simulink model "Waveformmodel"  (R2021a)
settings: Solver=FixedStepAuto  StartTime=0.0  StopTime=1  FixedStep=0.001  RelTol=1e-3
values from neighbouring files (symbols this model uses):
  Clamp1Amp = x(2)    [Opti_Clamp1.m]    (also in Opti_Clamp1_exp.m; Opti_Clamp2.m = 0; Opti_Clamp2_exp.m = 0; Opti_ClampsSine.m = 0)
  Clamp1Width = x(1)    [Opti_Clamp1.m]    (also in Opti_Clamp1_exp.m; Opti_ClampsSine.m = 0.001; Opti_Shears.m = 0.001; Opti_fit_exp.m = 0.001)
  Clamp2Amp = 0    [Opti_Clamp1.m]    (also in Opti_Clamp1_exp.m; Opti_ClampsSine.m; Opti_ClampsSine_exp.m; Opti_Shears.m)
  Clamp2Width = 0.001    [Opti_Clamp1.m]    (also in Opti_Clamp1_exp.m; Opti_ClampsSine_exp.m; Opti_Shears_exp.m; Opti_fit_exp.m)
  ClampsSineAmp = 0    [Opti_Clamp1.m]    (also in Opti_Clamp1_exp.m; Opti_Clamp2.m; Opti_Clamp2_exp.m; Opti_Shears.m)
  ClampsSineWidth = 0.001    [Opti_Clamp1.m]    (also in Opti_Clamp1_exp.m; Opti_Clamp2.m; Opti_Clamp2_exp.m; Opti_Shears.m)
  pAmpGain = 1./[25, 25, 7.5, 7.5]    [Main.m]    (also in Opti_Clamp1.m; Opti_Clamp1_exp.m; Opti_clamp05pi.m; Opti_fit_exp.m)
  pClampAmpl = (pClampMax - pClampMin) / 2    (= 45)    [Main.m]    (also in Opti_Clamp1.m; Opti_Clamp1_exp.m; Opti_clamp05pi.m; Opti_fit_exp.m)
  pClampOffs = (pClampMax + pClampMin) / 2    (= 15)    [Main.m]    (also in Opti_Clamp.m = (pClampMax + pClampMin) / 2; Opti_Clamp1.m; Opti_Clamp1_exp.m; Opti_Clamp2.m = (pClampMax + pClampMin) / 2)
  pClampSatMax = 60    [Main.m]    (also in Opti_Clamp.m; Opti_Clamp1.m; Opti_Clamp1_exp.m; Opti_Clamp2.m)
  pClampSatMin = -30    [Main.m]    (also in Opti_Clamp1.m; Opti_Clamp1_exp.m; Opti_clamp05pi.m; Opti_fit_exp.m)
  pShearAmpl = (pShearMax - pShearMin) / 2    (= 150)    [Main.m]    (also in Opti_Clamp1.m; Opti_Clamp1_exp.m; Opti_clamp05pi.m; Opti_fit_exp.m)
  pShearOffs = (pShearMax + pShearMin) / 2    (= 0)    [Main.m]    (also in Opti_Clamp.m = (pShearMax + pShearMin) / 2; Opti_Clamp1.m; Opti_Clamp1_exp.m; Opti_Clamp2.m = (pShearMax + pShearMin) / 2)
  pShearSatMax = 250    [Main.m]    (also in Opti_Clamp.m; Opti_Clamp1.m; Opti_Clamp1_exp.m; Opti_Clamp2.m)
  pShearSatMin = -250    [Main.m]    (also in Opti_Clamp1.m; Opti_Clamp1_exp.m; Opti_clamp05pi.m; Opti_fit_exp.m)
  ShearAmp = 0    [Opti_Clamp1.m]    (also in Opti_Clamp1_exp.m; Opti_Clamp2.m; Opti_Clamp2_exp.m; Opti_ClampsSine.m)
  ShearWidth = 0.001    [Opti_Clamp1.m]    (also in Opti_Clamp1_exp.m; Opti_Clamp2.m; Opti_Clamp2_exp.m; Opti_ClampsSine.m)
libraries: simulink x2
settings Model: Creator=20191779  LastModifiedBy=20191779

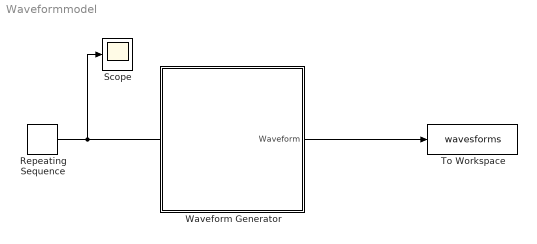
== system Waveformmodel ==
  Repeating Sequence : simulink/Sources/Repeating Sequence  rep_seq_t=[0 1 2]  rep_seq_y=[0 5 0]*5e-6
  Scope : Scope
  To Workspace : ToWorkspace  VariableName=wavesforms  SampleTime=-1
  Waveform Generator : Subsystem
  wires:
  Repeating Sequence/1 -> Scope/1
  Waveform Generator/1(Waveform) -> To Workspace/1

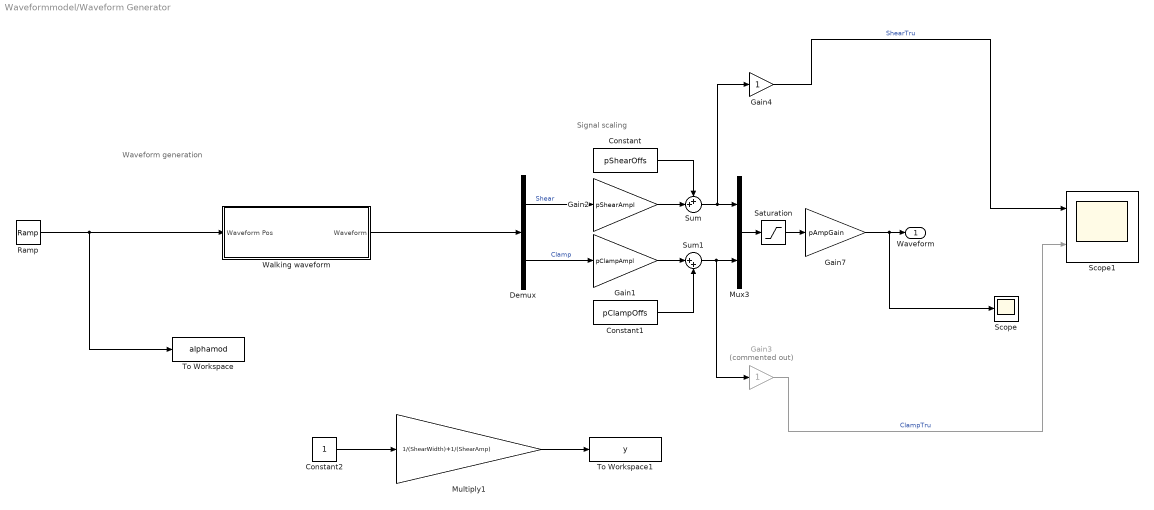
== system Waveformmodel/Waveform Generator ==
  note: Waveform generation
  note: Signal scaling
  Constant : Constant  Value=pShearOffs
  Constant1 : Constant  Value=pClampOffs
  Constant2 : Constant
  Demux : Demux  Outputs=2
  Gain1 : Gain  Gain=pClampAmpl
  Gain2 : Gain  Gain=pShearAmpl
  Gain3 : Gain  Commented=on
  Gain4 : Gain
  Gain7 : Gain  Gain=pAmpGain
  Multiply1 : Gain  Gain=1/(ShearWidth)+1/(ShearAmp)
  Mux3 : Mux  Inputs=2
  Ramp : simulink/Sources/Ramp  slope=2*pi  start=0  InitialOutput=0
  Saturation : Saturate  UpperLimit=[pShearSatMax pShearSatMax pClampSatMax pClampSatMax]  LowerLimit=[pShearSatMin pShearSatMin pClampSatMin pClampSatMin]
  Scope : Scope
  Scope1 : Scope  NumInputPorts=2
  Sum : Sum  Inputs=++|
  Sum1 : Sum  Inputs=|++
  To Workspace : ToWorkspace  VariableName=alphamod  SampleTime=-1
  To Workspace1 : ToWorkspace  VariableName=y  SampleTime=-1
  Walking waveform : Subsystem  TreatAsAtomicUnit=on
  Waveform : Outport  VectorParamsAs1DForOutWhenUnconnected=off
  wires:
  Gain2/1 -> Sum/2
  Constant/1 -> Sum/1
  Gain1/1 -> Sum1/1
  Constant1/1 -> Sum1/2
  Demux/1 -> Gain2/1  "Shear"
  Demux/2 -> Gain1/1  "Clamp"
  Gain3/1 -> Scope1/2  "ClampTru"
  Gain4/1 -> Scope1/1  "ShearTru"
  Walking waveform/1(Waveform) -> Demux/1
  Mux3/1 -> Saturation/1
  Gain7/1 -> Scope/1, Waveform/1
  Sum/1 -> Gain4/1, Mux3/1
  Sum1/1 -> Gain3/1, Mux3/2
  Saturation/1 -> Gain7/1
  Ramp/1 -> To Workspace/1, Walking waveform/1(Waveform Pos)
  Constant2/1 -> Multiply1/1
  Multiply1/1 -> To Workspace1/1

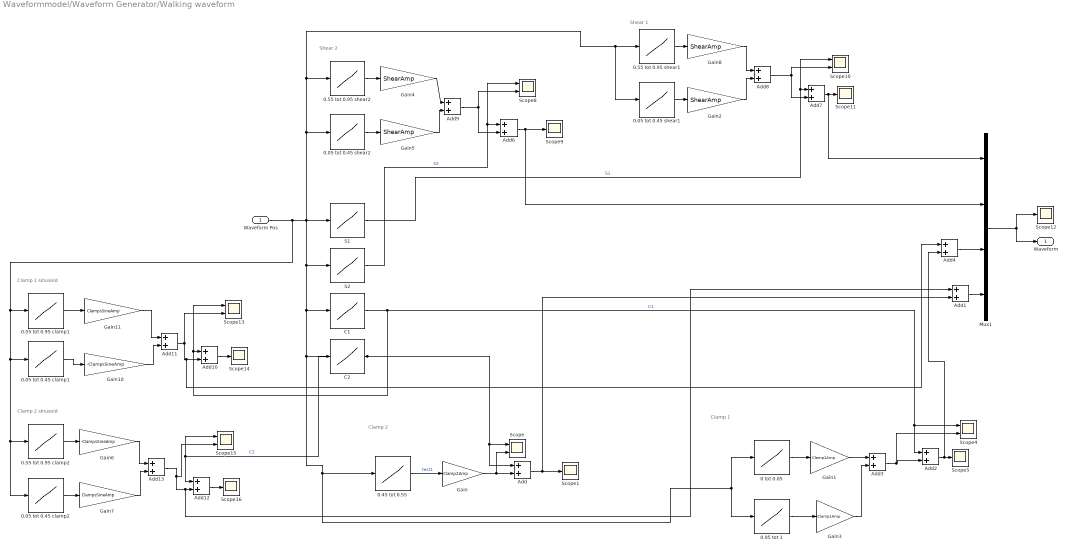
== system Waveformmodel/Waveform Generator/Walking waveform ==
  note: Shear 1
  note: Shear 2
  note: Clamp 2
  note: Clamp 1
  note: Clamp 1 sinusoid
  note: Clamp 2 sinusoid
  Waveform Pos : Inport
  0 tot 0.05 : Lookup_n-D  NumberOfTableDimensions=1  BreakpointsForDimension1="[(0.5-(Clamp1Width/2))*2*pi, 0.5*2*pi,  (0.5+(Clamp1Width/2))*2*pi]-pi"  Table=[0, -1, 0]  InterpMethod=Cubic spline  ExtrapMethod=Clip  InternalRulePriority=Speed  RndMeth=Simplest  InputSameDT=on
  0.05 tot 0.45 clamp1 : Lookup_n-D  NumberOfTableDimensions=1  BreakpointsForDimension1="[(0.5-ClampsSineWidth)*2*pi, ((0.5-ClampsSineWidth)+ClampsSineWidth/4)*2*pi,  ((0.5-ClampsSineWidth)+ClampsSineWidth/4*2)*2*pi,   ((0.5-ClampsSineWidth)+ClampsSineWidth/4*3)*2*pi,  ((0.5-ClampsSineWidth)+ClampsSineWidth)*2*pi]"  Table=[0, 1, 0, -1, 0]  InterpMethod=Cubic spline  ExtrapMethod=Clip  InternalRulePriority=Speed  RndMeth=Simplest  InputSameDT=on
  0.05 tot 0.45 clamp2 : Lookup_n-D  NumberOfTableDimensions=1  BreakpointsForDimension1="[(0.5-ClampsSineWidth)*2*pi, ((0.5-ClampsSineWidth)+ClampsSineWidth/4)*2*pi,  ((0.5-ClampsSineWidth)+ClampsSineWidth/4*2)*2*pi,   ((0.5-ClampsSineWidth)+ClampsSineWidth/4*3)*2*pi,  ((0.5-ClampsSineWidth)+ClampsSineWidth)*2*pi]"  Table=[0, 1, 0, -1, 0]  InterpMethod=Cubic spline  ExtrapMethod=Clip  InternalRulePriority=Speed  RndMeth=Simplest  InputSameDT=on
  0.05 tot 0.45 shear1 : Lookup_n-D  NumberOfTableDimensions=1  BreakpointsForDimension1="[(0.5-ShearWidth)*2*pi, ((0.5-ShearWidth)+ShearWidth/4)*2*pi,  ((0.5-ShearWidth)+ShearWidth/4*2)*2*pi,   ((0.5-ShearWidth)+ShearWidth/4*3)*2*pi,  ((0.5-ShearWidth)+ShearWidth)*2*pi]"  Table=[0, 1, 0, -1, 0]  InterpMethod=Cubic spline  ExtrapMethod=Clip  InternalRulePriority=Speed  RndMeth=Simplest  InputSameDT=on
  0.05 tot 0.45 shear2 : Lookup_n-D  NumberOfTableDimensions=1  BreakpointsForDimension1="[(0.5-ShearWidth)*2*pi, ((0.5-ShearWidth)+ShearWidth/4)*2*pi,  ((0.5-ShearWidth)+ShearWidth/4*2)*2*pi,   ((0.5-ShearWidth)+ShearWidth/4*3)*2*pi,  ((0.5-ShearWidth)+ShearWidth)*2*pi]"  Table=[0, 1, 0, -1, 0]  InterpMethod=Cubic spline  ExtrapMethod=Clip  InternalRulePriority=Speed  RndMeth=Simplest  InputSameDT=on
  0.45 tot 0.55 : Lookup_n-D  NumberOfTableDimensions=1  BreakpointsForDimension1="[(0.5-(Clamp2Width/2))*2*pi, 0.5*2*pi,  (0.5+(Clamp2Width/2))*2*pi]"  Table=[0, -1, 0]  InterpMethod=Cubic spline  ExtrapMethod=Clip  InternalRulePriority=Speed  RndMeth=Simplest  InputSameDT=on
  0.55 tot 0.95 clamp1 : Lookup_n-D  NumberOfTableDimensions=1  BreakpointsForDimension1="[(0.5-ClampsSineWidth)*2*pi, ((0.5-ClampsSineWidth)+ClampsSineWidth/4)*2*pi,  ((0.5-ClampsSineWidth)+ClampsSineWidth/4*2)*2*pi,   ((0.5-ClampsSineWidth)+ClampsSineWidth/4*3)*2*pi,  ((0.5-ClampsSineWidth)+ClampsSineWidth)*2*pi]+pi"  Table=[0, 1, 0, -1, 0]  InterpMethod=Cubic spline  ExtrapMethod=Clip  InternalRulePriority=Speed  RndMeth=Simplest  InputSameDT=on
  0.55 tot 0.95 clamp2 : Lookup_n-D  NumberOfTableDimensions=1  BreakpointsForDimension1="[(0.5-ClampsSineWidth)*2*pi, ((0.5-ClampsSineWidth)+ClampsSineWidth/4)*2*pi,  ((0.5-ClampsSineWidth)+ClampsSineWidth/4*2)*2*pi,   ((0.5-ClampsSineWidth)+ClampsSineWidth/4*3)*2*pi,  ((0.5-ClampsSineWidth)+ClampsSineWidth)*2*pi]+pi"  Table=[0, 1, 0, -1, 0]  InterpMethod=Cubic spline  ExtrapMethod=Clip  InternalRulePriority=Speed  RndMeth=Simplest  InputSameDT=on
  0.55 tot 0.95 shear1 : Lookup_n-D  NumberOfTableDimensions=1  BreakpointsForDimension1="[(0.5-ShearWidth)*2*pi, ((0.5-ShearWidth)+ShearWidth/4)*2*pi,  ((0.5-ShearWidth)+ShearWidth/4*2)*2*pi,   ((0.5-ShearWidth)+ShearWidth/4*3)*2*pi,  ((0.5-ShearWidth)+ShearWidth)*2*pi]+pi"  Table=[0, 1, 0, -1, 0]  InterpMethod=Cubic spline  ExtrapMethod=Clip  InternalRulePriority=Speed  RndMeth=Simplest  InputSameDT=on
  0.55 tot 0.95 shear2 : Lookup_n-D  NumberOfTableDimensions=1  BreakpointsForDimension1="[(0.5-ShearWidth)*2*pi, ((0.5-ShearWidth)+ShearWidth/4)*2*pi,  ((0.5-ShearWidth)+ShearWidth/4*2)*2*pi,   ((0.5-ShearWidth)+ShearWidth/4*3)*2*pi,  ((0.5-ShearWidth)+ShearWidth)*2*pi]+pi"  Table=[0, 1, 0, -1, 0]  InterpMethod=Cubic spline  ExtrapMethod=Clip  InternalRulePriority=Speed  RndMeth=Simplest  InputSameDT=on
  0.95 tot 1 : Lookup_n-D  NumberOfTableDimensions=1  BreakpointsForDimension1="[(0.5-(Clamp1Width/2))*2*pi, 0.5*2*pi,  (0.5+(Clamp1Width/2))*2*pi]+pi"  Table=[0, -1, 0]  InterpMethod=Cubic spline  ExtrapMethod=Clip  InternalRulePriority=Speed  RndMeth=Simplest  InputSameDT=on
  Add{,1..4,6..13} (13 alike) : Sum
  C1 : Lookup_n-D  NumberOfTableDimensions=1  BreakpointsForDimension1=[0, 0.05*2*pi, 0.45*2*pi, 0.55*2*pi, 0.95*2*pi, 1*2*pi]  Table=[1, 1, -1, -1, 1, 1]  InternalRulePriority=Speed  RndMeth=Simplest  InputSameDT=on
  C2 : Lookup_n-D  NumberOfTableDimensions=1  BreakpointsForDimension1=[0, 0.05*2*pi, 0.45*2*pi, 0.55*2*pi, 0.95*2*pi, 1*2*pi]  Table=[-1, -1, 1, 1, -1, -1]  InternalRulePriority=Speed  RndMeth=Simplest  InputSameDT=on
  Gain : Gain  Gain=Clamp2Amp
  Gain1 : Gain  Gain=Clamp1Amp
  Gain10 : Gain  Gain=-ClampsSineAmp
  Gain11 : Gain  Gain=ClampsSineAmp
  Gain{2,4..5,8} (4 alike) : Gain  Gain=ShearAmp
  Gain3 : Gain  Gain=Clamp1Amp
  Gain6 : Gain  Gain=-ClampsSineAmp
  Gain7 : Gain  Gain=ClampsSineAmp
  Mux1 : Mux
  S1 : Lookup_n-D  NumberOfTableDimensions=1  BreakpointsForDimension1=[0, 0.45*2*pi, 0.55*2*pi, 1*2*pi]  Table=[0, 1, -1, 0]  InternalRulePriority=Speed  RndMeth=Simplest  InputSameDT=on
  S2 : Lookup_n-D  NumberOfTableDimensions=1  BreakpointsForDimension1=[0, 0.05*2*pi, 0.95*2*pi, 1*2*pi]  Table=[0, -1, 1, 0]  InternalRulePriority=Speed  RndMeth=Simplest  InputSameDT=on
  Scope{,4,8,10,13,15} (6 alike) : Scope  NumInputPorts=2
  Scope{1,5,9,11..12,14,16} (7 alike) : Scope
  Waveform : Outport  VectorParamsAs1DForOutWhenUnconnected=off
  wires:
  Mux1/1 -> Waveform/1, Scope12/1
  0.45 tot 0.55/1 -> Gain/1  "test1"
  Gain/1 -> Add/2, Scope/2
  Add/1 -> Add1/2, Scope1/1
  Add2/1 -> Add4/2, Scope5/1
  0.95 tot 1/1 -> Gain3/1
  Gain1/1 -> Add3/1
  Add3/1 -> Add2/2, Scope4/2
  Gain3/1 -> Add3/2
  Add6/1 -> Mux1/2, Scope9/1
  S2/1 -> Scope8/1, Add6/1  "S2"
  0.05 tot 0.45 shear2/1 -> Gain5/1
  S1/1 -> Scope10/1, Add7/1  "S1"
  Add7/1 -> Mux1/1, Scope11/1
  Gain2/1 -> Add8/2
  0.55 tot 0.95 shear1/1 -> Gain8/1
  Add8/1 -> Add7/2, Scope10/2
  Gain8/1 -> Add8/1
  0.55 tot 0.95 shear2/1 -> Gain4/1
  Gain5/1 -> Add9/2
  Gain4/1 -> Add9/1
  Add9/1 -> Add6/2, Scope8/2
  Gain11/1 -> Add11/1
  Gain10/1 -> Add11/2
  Add11/1 -> Scope13/2, Add4/1, Add10/2
  Add10/1 -> Scope14/1
  C1/1 -> Scope13/1, Add10/1, Add2/1, Scope4/1  "C1"
  0.05 tot 0.45 clamp1/1 -> Gain10/1
  0.55 tot 0.95 clamp1/1 -> Gain11/1
  Waveform Pos/1 -> 0.05 tot 0.45 clamp2/1, 0.55 tot 0.95 clamp2/1, 0.05 tot 0.45 clamp1/1, 0.55 tot 0.95 clamp1/1, 0.55 tot 0.95 shear2/1, 0.05 tot 0.45 shear1/1, 0.55 tot 0.95 shear1/1, 0.05 tot 0.45 shear2/1, C2/1, 0.95 tot 1/1, 0 tot 0.05/1, 0.45 tot 0.55/1, C1/1, S2/1, S1/1
  Gain6/1 -> Add13/1
  Add12/1 -> Scope16/1
  0.55 tot 0.95 clamp2/1 -> Gain6/1
  0.05 tot 0.45 clamp2/1 -> Gain7/1
  Add13/1 -> Add1/1, Add12/2, Scope15/2
  C2/1 -> Scope/1, Add/1, Add12/1, Scope15/1  "C2"
  Gain7/1 -> Add13/2
  0 tot 0.05/1 -> Gain1/1
  0.05 tot 0.45 shear1/1 -> Gain2/1
  Add1/1 -> Mux1/4
  Add4/1 -> Mux1/3
